simulink model "Fig315"  (R2014b)
settings: Solver=ode3  StartTime=0.0  StopTime=10.007  FixedStep=2e-6  RelTol=1e-5
libraries: commutil2 x2, commfilt2 x1, commchan3 x1, commsink2 x1, commrandsrc2 x1
settings Model: Creator=Dennis Silage  LastModifiedBy=Silage
settings DataIOCC: SignalLoggingSaveFormat=ModelDataLogs
settings OptimizationCC: ExpressionDepthLimit=2147483647  InitFltsAndDblsToZero=on
settings DebuggingCC: UnderspecifiedInitializationDetection=Classic  MergeDetectMultiDrivingBlocksExec=none  SolverPrmCheckMsg=none  FcnCallInpInsideContextMsg=UseLocalSettings  StateNameClashWarn=warning
settings GRTTargetCC: CombineOutputUpdateFcns=off  GRTInterface=on

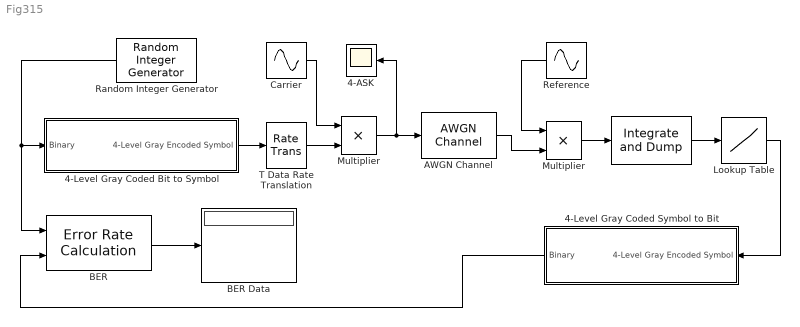
== system Fig315 ==
  " " : commfilt2/Integrate and Dump  obssamples=1000  offsetsamples=0  nodump=off  roundingMode=Floor  overflowMode=off
  4-ASK : Scope
      settings: YMin=-6  YMax=6  SaveName=ScopeData3
  4-Level Gray Coded Bit to Symbol : Subsystem
  4-Level Gray Coded Symbol to Bit : Subsystem
  AWGN Channel : commchan3/AWGN Channel  InputProcessing=Inherited (this choice will be removed - see release notes)  seed=randseed  noiseMode="Signal to noise ratio  (Eb/No)"  EbNodB=60  EsNodB=20  SNRdB=10  bitsPerSym=2  Ps=4.86  Tsym=2e-3  variance=0
  BER : commsink2/Error Rate Calculation  N=8  st_delay=0  cp_mode=Entire frame  subframe=[]  PMode=Port  WsName=ErrorVec  RsMode2=off  stop=off  numErr=100  maxBits=1e6
  BER Data : Display
  Carrier : Sin  Amplitude=1.66666  Frequency=40000*pi  SampleTime=2e-6
  Lookup Table : Lookup_n-D  NumberOfTableDimensions=1  BreakpointsForDimension1=[0, 4166.666, 8333.333, 12500]  BreakpointsForDimension3=[5, 7]  BreakpointsForDimension1DataTypeStr=double  Table=[0, 1, 2, 3]  TableDataTypeStr=double  InterpMethod=Nearest  InternalRulePriority=Speed  OutDataTypeStr=double  RndMeth=Simplest
  Multiplier : Product  RndMeth=Zero
  "Multiplier " : Product  RndMeth=Zero
  Random Integer Generator : commrandsrc2/Random Integer Generator  mul=2  seed=37  Ts=1e-3  frameBased=off  sampPerFrame=1  orient=off  outDataType=double
  Reference : Sin  Amplitude=5  Frequency=40000*pi  SampleTime=2e-6
  T Data Rate Translation : RateTransition  OutPortSampleTime=2e-6
  wires:
  BER/1 -> BER Data/1
  Multiplier/1 -> " "/1
  Random Integer Generator/1 -> 4-Level Gray Coded Bit to Symbol/1(Binary), BER/1
  "Multiplier "/1 -> AWGN Channel/1, 4-ASK/1
  Carrier/1 -> "Multiplier "/1
  4-Level Gray Coded Bit to Symbol/1(4-Level Gray Encoded Symbol) -> T Data Rate Translation/1
  T Data Rate Translation/1 -> "Multiplier "/2
  Reference/1 -> Multiplier/1
  AWGN Channel/1 -> Multiplier/2
  Lookup Table/1 -> 4-Level Gray Coded Symbol to Bit/1(4-Level Gray Encoded Symbol)
  " "/1 -> Lookup Table/1
  4-Level Gray Coded Symbol to Bit/1(Binary) -> BER/2

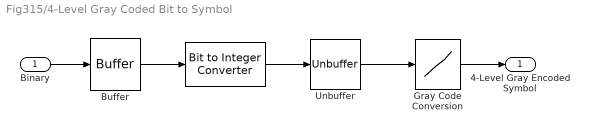
== system Fig315/4-Level Gray Coded Bit to Symbol ==
  Binary : Inport
  " " : commutil2/Bit to Integer Converter  nbits=2  bitOrder=MSB first  signedOutputValues=Unsigned  outDtype=Inherit via internal rule  outDtypeSigned=Inherit via internal rule
  Buffer : Buffer  N=2  TreatMby1Signals=One channel
  Gray Code Conversion : Lookup_n-D  NumberOfTableDimensions=1  BreakpointsForDimension1=[0, 1, 2, 3]  BreakpointsForDimension3=[5, 7]  BreakpointsForDimension1DataTypeStr=double  IndexSearchMethod=Linear search  Table=[0, 1, 3, 2]  TableDataTypeStr=double  InternalRulePriority=Speed  OutDataTypeStr=double  RndMeth=Simplest  InputSameDT=on
  Unbuffer : Unbuffer  SampleBasedProcessing=Same as frame based
  4-Level Gray Encoded Symbol : Outport
  wires:
  Gray Code Conversion/1 -> 4-Level Gray Encoded Symbol/1
  Binary/1 -> Buffer/1
  Buffer/1 -> " "/1
  " "/1 -> Unbuffer/1
  Unbuffer/1 -> Gray Code Conversion/1

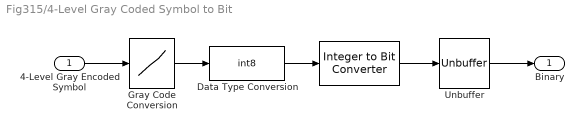
== system Fig315/4-Level Gray Coded Symbol to Bit ==
  4-Level Gray Encoded Symbol : Inport
  " " : commutil2/Integer to Bit Converter  nbits=2  signedInputValues=Unsigned  bitOrder=MSB first  outDtype=double
  Data Type Conversion : DataTypeConversion  OutDataTypeStr=int8  RndMeth=Nearest
  Gray Code Conversion : Lookup_n-D  NumberOfTableDimensions=1  BreakpointsForDimension1=[0, 1, 2, 3]  BreakpointsForDimension3=[5, 7]  BreakpointsForDimension1DataTypeStr=double  IndexSearchMethod=Linear search  Table=[0, 1, 3, 2]  TableDataTypeStr=double  InternalRulePriority=Speed  OutDataTypeStr=double  RndMeth=Simplest  InputSameDT=on
  Unbuffer : Unbuffer  SampleBasedProcessing=Same as frame based
  Binary : Outport
  wires:
  " "/1 -> Unbuffer/1
  4-Level Gray Encoded Symbol/1 -> Gray Code Conversion/1
  Unbuffer/1 -> Binary/1
  Data Type Conversion/1 -> " "/1
  Gray Code Conversion/1 -> Data Type Conversion/1
